simulink model "RE35_2019a"  (R2019a)
settings: Solver=VariableStepAuto  StartTime=0.0  StopTime=T_E  MaxStep=D_t  RelTol=1e-3
values from neighbouring files (symbols this model uses):
  J = 6.81e-6    (= 6.81e-06)    [DC_contr_ZN.m]    (also in DC_mot_TF.m; RE_35.m)
  K_b = 0.0388    [DC_contr_ZN.m]    (also in DC_mot_TF.m; Maxon_Control_BD.m = 0.0388182788029; RE_35.m)
  K_f = 6.33e-6    (= 6.33e-06)    [DC_contr_ZN.m]    (also in DC_mot_TF.m; Kf.m = 6.33589917605e-06; Maxon_Control_BD.m = 4.80152536515e-06; RE_35.m = Kf)
  K_m = 0.0389    [DC_contr_ZN.m]    (also in DC_mot_TF.m; Kf.m; Maxon_Control_BD.m; RE_35.m)
  Ki = contr_param (1)    [Maxon_Control_BD.m]    (also in RE_35.m = 256.41025641; pole_place.m = double(sol.Ki))
  Kp = contr_param (2)    [Maxon_Control_BD.m]    (also in RE_35.m = 82.8; pole_place.m = double(sol.Kp))
  L = 0.34e-3    (= 0.00034)    [DC_contr_ZN.m]    (also in DC_mot_TF.m; RE_35.m)
  N = 10e3    (= 10000)    [RE_35.m]
  R = 1.2    [DC_contr_ZN.m]    (also in DC_mot_TF.m; RE_35.m)
  T_e = 0.08    [RE_35.m]
  T_nom = 0.0972    [DC_contr_ZN.m]    (also in DC_mot_TF.m; Maxon_Control_BD.m = 0.101; RE_35.m)
  Td = T_crit/8    (= 0.000975)    [RE_35.m]
libraries: simulink x2
settings Model: Creator=manfred  LastModifiedBy=manfred

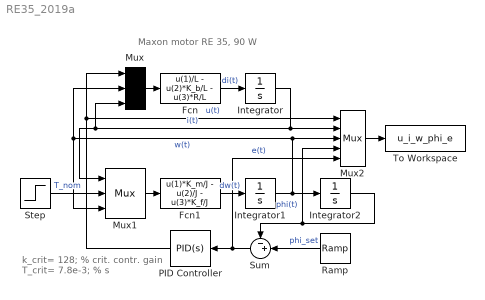
== system RE35_2019a ==
  note: k_crit= 128;      % crit. contr. gain
      | T_crit= 7.8e-3;  % s
  note: Maxon motor RE 35, 90 W
  Fcn : Fcn  Expr=u(1)/L - u(2)*K_b/L - u(3)*R/L
  Fcn1 : Fcn  Expr=u(1)*K_m/J - u(2)/J - u(3)*K_f/J
  Integrator : Integrator  ContinuousStateAttributes='i'
  Integrator1 : Integrator
  Integrator2 : Integrator
  Mux : Mux  Inputs=3
      settings: DisplayOption=signals
  Mux1 : Mux  Inputs=3
      settings: DisplayOption=signals
  Mux2 : Mux  Inputs=5
      settings: DisplayOption=signals
  PID Controller : simulink/Continuous/PID Controller  Controller=PID  Form=Ideal  TimeDomain=Continuous-time  SampleTime=-1  IntegratorMethod=Forward Euler  FilterMethod=Forward Euler  ControllerParametersSource=internal  P=Kp  I=Ki  D=Td  UseFilter=on  N=N  TunerSelectOption=Frequency Response Based  InitialConditionSource=internal  InitialConditionForIntegrator=0  InitialConditionForFilter=0  DifferentiatorICPrevScaledInput=0  ExternalReset=none  TrackingMode=off  Kt=1  LimitOutput=off  UpperSaturationLimit=inf  LowerSaturationLimit=-inf  LinearizeAsGain=on  AntiWindupMode=none  Kb=1  POutMin=[]  POutMax=[]  IOutMin=[]  IOutMax=[]  DOutMin=[]  DOutMax=[]  NOutMin=[]  NOutMax=[]  SumOutMin=[]  SumOutMax=[]  SaturationOutMin=[]  SaturationOutMax=[]  PParamMin=[]  PParamMax=[]  IParamMin=[]  IParamMax=[]  DParamMin=[]  DParamMax=[]  NParamMin=[]  NParamMax=[]  KbParamMin=[]  KbParamMax=[]  KtParamMin=[]  KtParamMax=[]  KbOutMin=[]  KbOutMax=[]  KtOutMin=[]  KtOutMax=[]  IntegratorOutMin=[]  IntegratorOutMax=[]  FilterOutMin=[]  FilterOutMax=[]  SumI1OutMin=[]  SumI1OutMax=[]  SumI2OutMin=[]  SumI2OutMax=[]  SumI3OutMin=[]  SumI3OutMax=[]  SumI4OutMin=[]  SumI4OutMax=[]  SumDOutMin=[]  SumDOutMax=[]  DifferentiatorOutMin=[]  DifferentiatorOutMax=[]  FilterDiffOutCoefMin=[]  FilterDiffOutCoefMax=[]  ReciprocalOutMin=[]  ReciprocalOutMax=[]  SumDenOutMin=[]  SumDenOutMax=[]  SumNumOutMin=[]  SumNumOutMax=[]  DivideOutMin=[]  DivideOutMax=[]  IntegratorContinuousStateAttributes=''  IntegratorStateMustResolveToSignalObject=off  IntegratorRTWStateStorageClass=Auto  FilterContinuousStateAttributes=''  FilterStateMustResolveToSignalObject=off  FilterRTWStateStorageClass=Auto  ParallelPVariant=Passthrough  IdealPVariant=InternalParameters  IVariant=InternalParameters  DVariant=InternalParameters  IntegratorVariant=Continuous  SatVariant=Disabled  AWVariant=Passthrough  PCopyVariant=Disabled  TRVariant=Disabled  FdbkBlocksVariant=Forward  IdealPFdbkVariant=Disabled  SatFdbkVariant=Disabled  DerivativeFilterVariant=ContFilter  NVariant=InternalParameters  NCopyVariant=Disabled  FilterICVariant=InternalICsFilter  IntegratorICVariant=InternalICs  ExternalResetVariant=Disabled  TRSumVariant=Passthrough  SumFdbkVariant=Disabled  SumVariant=Sum_PID
  Ramp : simulink/Sources/Ramp  slope=4*pi/T_e  start=0  InitialOutput=0
  Step : Step  Time=T_e/2  After=T_nom  SampleTime=0
  Sum : Sum  Inputs=-+|
  To Workspace : ToWorkspace  VariableName=u_i_w_phi_e  SaveFormat=Timeseries  SampleTime=-1
  wires:
  Fcn/1 -> Integrator/1  "di(t)"
  Mux/1 -> Fcn/1
  Integrator/1 -> Mux1/1, Mux/3, Mux2/2  "i(t)"
  Integrator1/1 -> Mux1/3, Mux/2, Mux2/3, Integrator2/1  "w(t)"
  Mux1/1 -> Fcn1/1
  Fcn1/1 -> Integrator1/1  "dw(t)"
  Step/1 -> Mux1/2  "T_nom"
  Mux2/1 -> To Workspace/1
  PID Controller/1 -> Mux2/1, Mux/1  "u(t)"
  Sum/1 -> Mux2/5, PID Controller/1  "e(t)"
  Ramp/1 -> Sum/2  "phi_set"
  Integrator2/1 -> Sum/1, Mux2/4  "phi(t)"
